simulink model "transientStability_R2014B_SLX"  (R2014b)
settings: Solver=ode4  SolverMode=SingleTasking  StartTime=0.0  StopTime=10  FixedStep=0.01  MaxStep=0.01  RelTol=1e-3  AbsTol=1e-2
undefined symbols (not defined in the file): j, mpc
(part 3 of 4)

== system transientStability_R2014B_SLX/Turbine system/Sped Gov_Hydro Turbine/DEMUXg2 ==
  In1 : Inport
  Dummy Zeros : Constant  Value=zeros(1,mpc.dynamicdata.extraVariables.nb-size(mpc.dynamicdata.turb_hydro,1))
  Mux1 : Mux  Inputs="[mpc.dynamicdata.extraVariables.nb-size(mpc.dynamicdata.turb_hydro,1)  size(mpc.dynamicdata.turb_hydro,1)]"
  Selector4 : Selector  InputPortWidth=mpc.dynamicdata.extraVariables.nb  IndexOptions=Index vector (dialog)  Indices=mpc.dynamicdata.gen_turbineParameters.hydro_turbineParameters.order_hydro  OutputSizes=1
  Out1 : Outport
  wires:
  Mux1/1 -> Selector4/1
  Dummy Zeros/1 -> Mux1/1
  Selector4/1 -> Out1/1
  In1/1 -> Mux1/2

== system transientStability_R2014B_SLX/Turbine system/Sped Gov_Hydro Turbine/Governer ==
  del WB : Inport
  Constant : Constant  Value=mpc.dynamicdata.gen_turbineParameters.hydro_turbineParameters.Pgv_ht0
  Gain : Gain  Gain=1-mpc.dynamicdata.gen_turbineParameters.hydro_turbineParameters.T2_ht./mpc.dynamicdata.gen_turbineParameters.hydro_turbineParameters.T1_ht  SaturateOnIntegerOverflow=on  OutDataTypeStr=Inherit: Same as input  ParamDataTypeStr=Inherit: Same as input
  Gain1 : Gain  Gain=1./mpc.dynamicdata.gen_turbineParameters.hydro_turbineParameters.T1_ht  SaturateOnIntegerOverflow=on  OutDataTypeStr=Inherit: Same as input  ParamDataTypeStr=Inherit: Same as input
  Gain2 : Gain  Gain=mpc.dynamicdata.gen_turbineParameters.hydro_turbineParameters.T2_ht./mpc.dynamicdata.gen_turbineParameters.hydro_turbineParameters.T1_ht  SaturateOnIntegerOverflow=on  OutDataTypeStr=Inherit: Same as input  ParamDataTypeStr=Inherit: Same as input
  Gain3 : Gain  Gain=mpc.dynamicdata.gen_turbineParameters.hydro_turbineParameters.K_ht  SaturateOnIntegerOverflow=on  OutDataTypeStr=Inherit: Same as input  ParamDataTypeStr=Inherit: Same as input
  Gain4 : Gain  Gain=1./mpc.dynamicdata.gen_turbineParameters.hydro_turbineParameters.T3_ht  SaturateOnIntegerOverflow=on  OutDataTypeStr=Inherit: Same as input  ParamDataTypeStr=Inherit: Same as input
  Integrator : Integrator
  Integrator1 : Integrator
  Saturation : Saturate  UpperLimit=mpc.dynamicdata.gen_turbineParameters.hydro_turbineParameters.Pgv_ht_max.*mpc.dynamicdata.gen_turbineParameters.hydro_turbineParameters.Pgv_ht0  LowerLimit=mpc.dynamicdata.gen_turbineParameters.hydro_turbineParameters.Pgv_ht_min.*mpc.dynamicdata.gen_turbineParameters.hydro_turbineParameters.Pgv_ht0
  Sum : Sum  Inputs=+-  SaturateOnIntegerOverflow=on  InputSameDT=on  OutDataTypeStr=Inherit: Same as first input
  Sum1 : Sum  SaturateOnIntegerOverflow=on  InputSameDT=on  OutDataTypeStr=Inherit: Same as first input
  Sum3 : Sum  Inputs=+-  SaturateOnIntegerOverflow=on  InputSameDT=on  OutDataTypeStr=Inherit: Same as first input
  Sum4 : Sum  Inputs=+-  SaturateOnIntegerOverflow=on  InputSameDT=on  OutDataTypeStr=Inherit: Same as first input
  Pgv : Outport
  wires:
  Sum/1 -> Gain1/1
  Gain/1 -> Sum/1
  Integrator/1 -> Sum/2, Sum1/1
  Gain2/1 -> Sum1/2
  Gain1/1 -> Integrator/1
  del WB/1 -> Gain2/1, Gain/1
  Sum1/1 -> Gain3/1
  Gain3/1 -> Sum3/1
  Sum3/1 -> Gain4/1
  Gain4/1 -> Integrator1/1
  Integrator1/1 -> Sum4/2, Sum3/2
  Constant/1 -> Sum4/1
  Sum4/1 -> Saturation/1
  Saturation/1 -> Pgv/1

== system transientStability_R2014B_SLX/Turbine system/Sped Gov_Hydro Turbine/HydroTurbine ==
  Pgv : Inport
  Gain : Gain  Gain=1-(-mpc.dynamicdata.gen_turbineParameters.hydro_turbineParameters.T_wht)./(0.5*mpc.dynamicdata.gen_turbineParameters.hydro_turbineParameters.T_wht)  SaturateOnIntegerOverflow=on  OutDataTypeStr=Inherit: Same as input  ParamDataTypeStr=Inherit: Same as input
  Gain1 : Gain  Gain=1./(0.5*mpc.dynamicdata.gen_turbineParameters.hydro_turbineParameters.T_wht)  SaturateOnIntegerOverflow=on  OutDataTypeStr=Inherit: Same as input  ParamDataTypeStr=Inherit: Same as input
  Gain2 : Gain  Gain=-mpc.dynamicdata.gen_turbineParameters.hydro_turbineParameters.T_wht./(0.5*mpc.dynamicdata.gen_turbineParameters.hydro_turbineParameters.T_wht)  SaturateOnIntegerOverflow=on  OutDataTypeStr=Inherit: Same as input  ParamDataTypeStr=Inherit: Same as input
  Integrator : Integrator  InitialCondition=mpc.dynamicdata.gen_turbineParameters.hydro_turbineParameters.Tgr_ht0
  Sum : Sum  Inputs=+-  SaturateOnIntegerOverflow=on  InputSameDT=on  OutDataTypeStr=Inherit: Same as first input
  Sum1 : Sum  SaturateOnIntegerOverflow=on  InputSameDT=on  OutDataTypeStr=Inherit: Same as first input
  Tm : Outport
  wires:
  Sum1/1 -> Tm/1
  Gain1/1 -> Integrator/1
  Pgv/1 -> Gain2/1, Gain/1
  Gain2/1 -> Sum1/2
  Integrator/1 -> Sum/2, Sum1/1
  Gain/1 -> Sum/1
  Sum/1 -> Gain1/1

== system transientStability_R2014B_SLX/Turbine system/Sped Gov_Hydro Turbine/Select-Turbine ==
  in_1 : Inport
  in_2 : Inport  Port=2
  Switch : Switch  Threshold=1  SaturateOnIntegerOverflow=on  InputSameDT=on
  zeros : Constant  Value=zeros(1,mpc.dynamicdata.extraVariables.nb)
  out_1 : Outport  InitialOutput=0
  wires:
  Switch/1 -> out_1/1
  in_1/1 -> Switch/2
  in_2/1 -> Switch/3
  zeros/1 -> Switch/1

== system transientStability_R2014B_SLX/Turbine system/Speed Gov. Reheat Steam Turbine/DEMUXg2 ==
  In1 : Inport
  Dummy Zeros : Constant  Value=zeros(1,mpc.dynamicdata.extraVariables.nb-size(mpc.dynamicdata.turb_rhst,1))
  Mux1 : Mux  Inputs="[mpc.dynamicdata.extraVariables.nb-size(mpc.dynamicdata.turb_rhst,1)  size(mpc.dynamicdata.turb_rhst,1)]"
  Selector4 : Selector  InputPortWidth=mpc.dynamicdata.extraVariables.nb  IndexOptions=Index vector (dialog)  Indices=mpc.dynamicdata.gen_turbineParameters.Reheat_turbineParameters.order_rhst  OutputSizes=1
  Out1 : Outport
  wires:
  In1/1 -> Mux1/2
  Selector4/1 -> Out1/1
  Dummy Zeros/1 -> Mux1/1
  Mux1/1 -> Selector4/1

== system transientStability_R2014B_SLX/Turbine system/Speed Gov. Reheat Steam Turbine/Governer ==
  dWB : Inport
  Constant : Constant  Value=mpc.dynamicdata.gen_turbineParameters.Reheat_turbineParameters.Pgv_rht0
  Gain : Gain  Gain=1-mpc.dynamicdata.gen_turbineParameters.Reheat_turbineParameters.T2_rht./mpc.dynamicdata.gen_turbineParameters.Reheat_turbineParameters.T1_rht  SaturateOnIntegerOverflow=on  OutDataTypeStr=Inherit: Same as input  ParamDataTypeStr=Inherit: Same as input
  Gain1 : Gain  Gain=1./mpc.dynamicdata.gen_turbineParameters.Reheat_turbineParameters.T1_rht  SaturateOnIntegerOverflow=on  OutDataTypeStr=Inherit: Same as input  ParamDataTypeStr=Inherit: Same as input
  Gain2 : Gain  Gain=mpc.dynamicdata.gen_turbineParameters.Reheat_turbineParameters.T2_rht./mpc.dynamicdata.gen_turbineParameters.Reheat_turbineParameters.T1_rht  SaturateOnIntegerOverflow=on  OutDataTypeStr=Inherit: Same as input  ParamDataTypeStr=Inherit: Same as input
  Gain3 : Gain  Gain=mpc.dynamicdata.gen_turbineParameters.Reheat_turbineParameters.K_rht  SaturateOnIntegerOverflow=on  OutDataTypeStr=Inherit: Same as input  ParamDataTypeStr=Inherit: Same as input
  Gain4 : Gain  Gain=1./mpc.dynamicdata.gen_turbineParameters.Reheat_turbineParameters.T3_rht  SaturateOnIntegerOverflow=on  OutDataTypeStr=Inherit: Same as input  ParamDataTypeStr=Inherit: Same as input
  Integrator : Integrator
  Integrator1 : Integrator  InitialCondition=mpc.dynamicdata.gen_turbineParameters.Reheat_turbineParameters.Pgv_rht0  LimitOutput=on  UpperSaturationLimit=mpc.dynamicdata.gen_turbineParameters.Reheat_turbineParameters.Pgv_rht_max.*mpc.dynamicdata.gen_turbineParameters.Reheat_turbineParameters.Pgv_rht0  LowerSaturationLimit=mpc.dynamicdata.gen_turbineParameters.Reheat_turbineParameters.Pgv_rht_min.*mpc.dynamicdata.gen_turbineParameters.Reheat_turbineParameters.Pgv_rht0
  Sum : Sum  Inputs=+-  SaturateOnIntegerOverflow=on  InputSameDT=on  OutDataTypeStr=Inherit: Same as first input
  Sum1 : Sum  SaturateOnIntegerOverflow=on  InputSameDT=on  OutDataTypeStr=Inherit: Same as first input
  Sum3 : Sum  Inputs=+--  SaturateOnIntegerOverflow=on  InputSameDT=on  OutDataTypeStr=Inherit: Same as first input
  Pgv : Outport
  wires:
  Sum/1 -> Gain1/1
  Gain/1 -> Sum/1
  Integrator/1 -> Sum1/1, Sum/2
  Gain2/1 -> Sum1/2
  Gain1/1 -> Integrator/1
  Sum1/1 -> Gain3/1
  Sum3/1 -> Gain4/1
  Gain4/1 -> Integrator1/1
  Integrator1/1 -> Sum3/3, Pgv/1
  Gain3/1 -> Sum3/2
  Constant/1 -> Sum3/1
  dWB/1 -> Gain/1, Gain2/1

== system transientStability_R2014B_SLX/Turbine system/Speed Gov. Reheat Steam Turbine/Reheat ==
  Pgv : Inport
  Crossover : Subsystem
  Gain3 : Gain  Gain=mpc.dynamicdata.gen_turbineParameters.Reheat_turbineParameters.FHP_rht  SaturateOnIntegerOverflow=on  OutDataTypeStr=Inherit: Same as input  ParamDataTypeStr=Inherit: Same as input
  Gain4 : Gain  Gain=mpc.dynamicdata.gen_turbineParameters.Reheat_turbineParameters.FIP_rht  SaturateOnIntegerOverflow=on  OutDataTypeStr=Inherit: Same as input  ParamDataTypeStr=Inherit: Same as input
  Gain5 : Gain  Gain=mpc.dynamicdata.gen_turbineParameters.Reheat_turbineParameters.FLP_rht  SaturateOnIntegerOverflow=on  OutDataTypeStr=Inherit: Same as input  ParamDataTypeStr=Inherit: Same as input
  Reheater : Subsystem
  St.Chest : Subsystem
  Sum5 : Sum  Inputs=+++  SaturateOnIntegerOverflow=on  InputSameDT=on  OutDataTypeStr=Inherit: Same as first input
  Pm : Outport
  wires:
  Crossover/1(Out1) -> Gain5/1
  Reheater/1(Out1) -> Crossover/1(In1), Gain4/1
  St.Chest/1(Out1) -> Reheater/1(In1), Gain3/1
  Gain5/1 -> Sum5/3
  Gain4/1 -> Sum5/2
  Gain3/1 -> Sum5/1
  Sum5/1 -> Pm/1
  Pgv/1 -> St.Chest/1(In1)

== system transientStability_R2014B_SLX/Turbine system/Speed Gov. Reheat Steam Turbine/Select-Turbine ==
  in_1 : Inport
  in_2 : Inport  Port=2
  Switch : Switch  Threshold=1  SaturateOnIntegerOverflow=on  InputSameDT=on
  zeros : Constant  Value=zeros(1,mpc.dynamicdata.extraVariables.nb)
  out_1 : Outport  InitialOutput=0
  wires:
  Switch/1 -> out_1/1
  in_1/1 -> Switch/2
  in_2/1 -> Switch/3
  zeros/1 -> Switch/1

== system transientStability_R2014B_SLX/Excitation system/Exciter_AC1A /Exciter AC1A/ESS ==
  vfe : Inport
  Gain3 : Gain  Gain=1./mpc.dynamicdata.gen_exciterParameters.AC1A_exciterParameters.TF_AC1A  SaturateOnIntegerOverflow=on  OutDataTypeStr=Inherit: Same as input  ParamDataTypeStr=Inherit: Same as input
  Gain4 : Gain  Gain=mpc.dynamicdata.gen_exciterParameters.AC1A_exciterParameters.KF_AC1A  SaturateOnIntegerOverflow=on  OutDataTypeStr=Inherit: Same as input  ParamDataTypeStr=Inherit: Same as input
  Integrator4 : Integrator  InitialCondition=mpc.dynamicdata.gen_exciterParameters.AC1A_exciterParameters.Fst0_AC1A
  Sum3 : Sum  Inputs=+-  SaturateOnIntegerOverflow=on  InputSameDT=on  OutDataTypeStr=Inherit: Same as first input
  VF1 : Outport
  wires:
  vfe/1 -> Gain4/1
  Sum3/1 -> Gain3/1
  Gain4/1 -> Sum3/1
  Gain3/1 -> Integrator4/1, VF1/1
  Integrator4/1 -> Sum3/2

== system transientStability_R2014B_SLX/Excitation system/Exciter_AC1A /Exciter AC1A/Regulator ==
  Vin : Inport
  Gain : Gain  Gain=1./mpc.dynamicdata.gen_exciterParameters.AC1A_exciterParameters.TA_AC1A  SaturateOnIntegerOverflow=on  OutDataTypeStr=Inherit: Same as input  ParamDataTypeStr=Inherit: Same as input
  Gain1 : Gain  Gain=mpc.dynamicdata.gen_exciterParameters.AC1A_exciterParameters.kA_AC1A  SaturateOnIntegerOverflow=on  OutDataTypeStr=Inherit: Same as input  ParamDataTypeStr=Inherit: Same as input
  Integrator2 : Integrator  InitialCondition=mpc.dynamicdata.gen_exciterParameters.AC1A_exciterParameters.VR0_AC1A  LimitOutput=on  UpperSaturationLimit=mpc.dynamicdata.gen_exciterParameters.AC1A_exciterParameters.VAmax_AC1A  LowerSaturationLimit=mpc.dynamicdata.gen_exciterParameters.AC1A_exciterParameters.VAmin_AC1A
  Sum : Sum  Inputs=+-  SaturateOnIntegerOverflow=on  InputSameDT=on  OutDataTypeStr=Inherit: Same as first input
  VR : Outport
  wires:
  Sum/1 -> Gain/1
  Integrator2/1 -> VR/1, Sum/2
  Gain1/1 -> Sum/1
  Gain/1 -> Integrator2/1
  Vin/1 -> Gain1/1

== system transientStability_R2014B_SLX/Excitation system/Exciter_AC1A /Exciter AC1A/Subsystem1 ==
  VE : Inport
  IFD : Inport  Port=2
  Rec-Reg Curve : Subsystem
  Saturation : Subsystem
  FEX : Outport
  VFE : Outport  Port=2
  wires:
  Rec-Reg Curve/1(Fex) -> FEX/1
  Saturation/1(Vfe) -> VFE/1
  VE/1 -> Saturation/1(Ve), Rec-Reg Curve/2(Ve)
  IFD/1 -> Saturation/2(Ifd), Rec-Reg Curve/1(Ifd)

== system transientStability_R2014B_SLX/Excitation system/Exciter_AC1A /Exciter AC1A/TGR ==
  Ver : Inport
  Gain3 : Gain  Gain=1./mpc.dynamicdata.gen_exciterParameters.AC1A_exciterParameters.TB_AC1A  SaturateOnIntegerOverflow=on  OutDataTypeStr=Inherit: Same as input  ParamDataTypeStr=Inherit: Same as input
  Gain4 : Gain  Gain=mpc.dynamicdata.gen_exciterParameters.AC1A_exciterParameters.TC_AC1A./mpc.dynamicdata.gen_exciterParameters.AC1A_exciterParameters.TB_AC1A  SaturateOnIntegerOverflow=on  OutDataTypeStr=Inherit: Same as input  ParamDataTypeStr=Inherit: Same as input
  Gain5 : Gain  Gain=1-mpc.dynamicdata.gen_exciterParameters.AC1A_exciterParameters.TC_AC1A./mpc.dynamicdata.gen_exciterParameters.AC1A_exciterParameters.TB_AC1A  SaturateOnIntegerOverflow=on  OutDataTypeStr=Inherit: Same as input  ParamDataTypeStr=Inherit: Same as input
  Integrator4 : Integrator  InitialCondition=mpc.dynamicdata.gen_exciterParameters.AC1A_exciterParameters.Tgr0_AC1A
  Sum3 : Sum  SaturateOnIntegerOverflow=on  InputSameDT=on  OutDataTypeStr=Inherit: Same as first input
  Sum4 : Sum  Inputs=+-  SaturateOnIntegerOverflow=on  InputSameDT=on  OutDataTypeStr=Inherit: Same as first input
  Vtgr : Outport
  wires:
  Sum3/1 -> Vtgr/1
  Gain4/1 -> Sum3/2
  Integrator4/1 -> Sum3/1, Sum4/2
  Sum4/1 -> Gain3/1
  Gain5/1 -> Sum4/1
  Gain3/1 -> Integrator4/1
  Ver/1 -> Gain4/1, Gain5/1

== system transientStability_R2014B_SLX/Excitation system/Exciter_AC1A /Exciter AC1A/delay1 ==
  Vin : Inport
  Gain : Gain  Gain=1./mpc.dynamicdata.gen_exciterParameters.AC1A_exciterParameters.Tr_AC1A  SaturateOnIntegerOverflow=on  OutDataTypeStr=Inherit: Same as input  ParamDataTypeStr=Inherit: Same as input
  Integrator2 : Integrator  InitialCondition=mpc.dynamicdata.extraVariables.lfl(mpc.dynamicdata.exc_AC1A(:,1),2)
  Sum : Sum  Inputs=+-  SaturateOnIntegerOverflow=on  InputSameDT=on  OutDataTypeStr=Inherit: Same as first input
  Out1 : Outport
  wires:
  Vin/1 -> Sum/1
  Integrator2/1 -> Sum/2, Out1/1
  Sum/1 -> Gain/1
  Gain/1 -> Integrator2/1

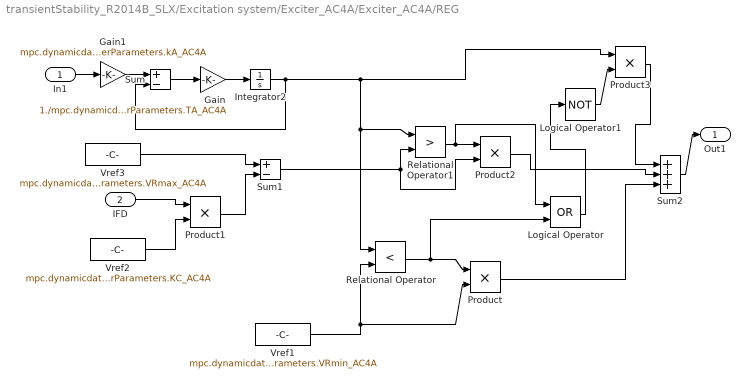
== system transientStability_R2014B_SLX/Excitation system/Exciter_AC4A/Exciter_AC4A/REG ==
  In1 : Inport
  IFD : Inport  Port=2
  Gain : Gain  Gain=1./mpc.dynamicdata.gen_exciterParameters.AC4A_exciterParameters.TA_AC4A  SaturateOnIntegerOverflow=on  OutDataTypeStr=Inherit: Same as input  ParamDataTypeStr=Inherit: Same as input
  Gain1 : Gain  Gain=mpc.dynamicdata.gen_exciterParameters.AC4A_exciterParameters.kA_AC4A  SaturateOnIntegerOverflow=on  OutDataTypeStr=Inherit: Same as input  ParamDataTypeStr=Inherit: Same as input
  Integrator2 : Integrator  InitialCondition=mpc.dynamicdata.gen_exciterParameters.AC4A_exciterParameters.Efd0_AC4A
  Logical Operator : Logic  Operator=OR
  Logical Operator1 : Logic  Operator=NOT
  Product{,1..3} (4 alike) : Product  SaturateOnIntegerOverflow=on  RndMeth=Zero  InputSameDT=on  OutDataTypeStr=Inherit: Same as first input
  Relational Operator : RelationalOperator  Operator=<  InputSameDT=on
  Relational Operator1 : RelationalOperator  Operator=>  InputSameDT=on
  Sum : Sum  Inputs=+-  SaturateOnIntegerOverflow=on  InputSameDT=on  OutDataTypeStr=Inherit: Same as first input
  Sum1 : Sum  Inputs=+-  SaturateOnIntegerOverflow=on  InputSameDT=on  OutDataTypeStr=Inherit: Same as first input
  Sum2 : Sum  Inputs=+++  SaturateOnIntegerOverflow=on  InputSameDT=on  OutDataTypeStr=Inherit: Same as first input
  Vref1 : Constant  Value=mpc.dynamicdata.gen_exciterParameters.AC4A_exciterParameters.VRmin_AC4A
  Vref2 : Constant  Value=mpc.dynamicdata.gen_exciterParameters.AC4A_exciterParameters.KC_AC4A
  Vref3 : Constant  Value=mpc.dynamicdata.gen_exciterParameters.AC4A_exciterParameters.VRmax_AC4A
  Out1 : Outport
  wires:
  In1/1 -> Gain1/1
  Gain1/1 -> Sum/1
  Sum/1 -> Gain/1
  Integrator2/1 -> Sum/2, Relational Operator/1, Relational Operator1/1, Product3/1
  Gain/1 -> Integrator2/1
  Vref1/1 -> Relational Operator/2, Product/2
  Vref2/1 -> Product1/2
  IFD/1 -> Product1/1
  Vref3/1 -> Sum1/1
  Product1/1 -> Sum1/2
  Sum1/1 -> Relational Operator1/2, Product2/2
  Product2/1 -> Sum2/2
  Product/1 -> Sum2/3
  Relational Operator/1 -> Product/1, Logical Operator/2
  Relational Operator1/1 -> Product2/1, Logical Operator/1
  Logical Operator/1 -> Logical Operator1/1
  Logical Operator1/1 -> Product3/2
  Product3/1 -> Sum2/1
  Sum2/1 -> Out1/1

== system transientStability_R2014B_SLX/Excitation system/Exciter_AC4A/Exciter_AC4A/TGR ==
  Ver : Inport
  Gain3 : Gain  Gain=1./mpc.dynamicdata.gen_exciterParameters.AC4A_exciterParameters.TB_AC4A  SaturateOnIntegerOverflow=on  OutDataTypeStr=Inherit: Same as input  ParamDataTypeStr=Inherit: Same as input
  Gain4 : Gain  Gain=mpc.dynamicdata.gen_exciterParameters.AC4A_exciterParameters.TC_AC4A./mpc.dynamicdata.gen_exciterParameters.AC4A_exciterParameters.TB_AC4A  SaturateOnIntegerOverflow=on  OutDataTypeStr=Inherit: Same as input  ParamDataTypeStr=Inherit: Same as input
  Gain5 : Gain  Gain=1-mpc.dynamicdata.gen_exciterParameters.AC4A_exciterParameters.TC_AC4A./mpc.dynamicdata.gen_exciterParameters.AC4A_exciterParameters.TB_AC4A  SaturateOnIntegerOverflow=on  OutDataTypeStr=Inherit: Same as input  ParamDataTypeStr=Inherit: Same as input
  Integrator4 : Integrator  InitialCondition=mpc.dynamicdata.gen_exciterParameters.AC4A_exciterParameters.Tgr0_AC4A
  Sum3 : Sum  SaturateOnIntegerOverflow=on  InputSameDT=on  OutDataTypeStr=Inherit: Same as first input
  Sum4 : Sum  Inputs=+-  SaturateOnIntegerOverflow=on  InputSameDT=on  OutDataTypeStr=Inherit: Same as first input
  V3 : Outport
  wires:
  Gain5/1 -> Sum4/1
  Sum4/1 -> Gain3/1
  Gain3/1 -> Integrator4/1
  Integrator4/1 -> Sum4/2, Sum3/1
  Gain4/1 -> Sum3/2
  Ver/1 -> Gain5/1, Gain4/1
  Sum3/1 -> V3/1

== system transientStability_R2014B_SLX/Excitation system/Exciter_AC4A/Exciter_AC4A/delay1 ==
  Vin : Inport
  Gain : Gain  Gain=1./mpc.dynamicdata.gen_exciterParameters.AC4A_exciterParameters.Tr_AC4A  SaturateOnIntegerOverflow=on  OutDataTypeStr=Inherit: Same as input  ParamDataTypeStr=Inherit: Same as input
  Integrator2 : Integrator  InitialCondition=mpc.dynamicdata.extraVariables.lfl(mpc.dynamicdata.exc_AC4A(:,1),2)
  Sum : Sum  Inputs=+-  SaturateOnIntegerOverflow=on  InputSameDT=on  OutDataTypeStr=Inherit: Same as first input
  Out1 : Outport
  wires:
  Vin/1 -> Sum/1
  Integrator2/1 -> Sum/2, Out1/1
  Sum/1 -> Gain/1
  Gain/1 -> Integrator2/1

== system transientStability_R2014B_SLX/Excitation system/Exciter_DC1A/Subsystem/ESS ==
  Efd : Inport
  Gain3 : Gain  Gain=1./mpc.dynamicdata.gen_exciterParameters.DC1A_exciterParameters.TF_DC1A  SaturateOnIntegerOverflow=on  OutDataTypeStr=Inherit: Same as input  ParamDataTypeStr=Inherit: Same as input
  Gain4 : Gain  Gain=mpc.dynamicdata.gen_exciterParameters.DC1A_exciterParameters.KF_DC1A  SaturateOnIntegerOverflow=on  OutDataTypeStr=Inherit: Same as input  ParamDataTypeStr=Inherit: Same as input
  Integrator4 : Integrator  InitialCondition=mpc.dynamicdata.gen_exciterParameters.DC1A_exciterParameters.Fst0_DC1A
  Sum3 : Sum  Inputs=+-  SaturateOnIntegerOverflow=on  InputSameDT=on  OutDataTypeStr=Inherit: Same as first input
  VF : Outport
  wires:
  Gain4/1 -> Sum3/1
  Sum3/1 -> Gain3/1
  Integrator4/1 -> Sum3/2
  Gain3/1 -> Integrator4/1, VF/1
  Efd/1 -> Gain4/1

== system transientStability_R2014B_SLX/Excitation system/Exciter_DC1A/Subsystem/Regulator ==
  Vin : Inport
  Gain : Gain  Gain=1./mpc.dynamicdata.gen_exciterParameters.DC1A_exciterParameters.TA_DC1A  SaturateOnIntegerOverflow=on  OutDataTypeStr=Inherit: Same as input  ParamDataTypeStr=Inherit: Same as input
  Gain1 : Gain  Gain=mpc.dynamicdata.gen_exciterParameters.DC1A_exciterParameters.KA_DC1A  SaturateOnIntegerOverflow=on  OutDataTypeStr=Inherit: Same as input  ParamDataTypeStr=Inherit: Same as input
  Integrator2 : Integrator  InitialCondition=mpc.dynamicdata.gen_exciterParameters.DC1A_exciterParameters.VR0_DC1A  LimitOutput=on  UpperSaturationLimit=mpc.dynamicdata.gen_exciterParameters.DC1A_exciterParameters.VRmax_DC1A  LowerSaturationLimit=mpc.dynamicdata.gen_exciterParameters.DC1A_exciterParameters.VRmin_DC1A
  Sum : Sum  Inputs=+-  SaturateOnIntegerOverflow=on  InputSameDT=on  OutDataTypeStr=Inherit: Same as first input
  Out1 : Outport
  wires:
  Gain1/1 -> Sum/1
  Integrator2/1 -> Sum/2, Out1/1
  Sum/1 -> Gain/1
  Gain/1 -> Integrator2/1
  Vin/1 -> Gain1/1

== system transientStability_R2014B_SLX/Excitation system/Exciter_DC1A/Subsystem/Saturation ==
  Efd : Inport
  Constant : Constant  Value=mpc.dynamicdata.gen_exciterParameters.DC1A_exciterParameters.B_DC1A
  Constant1 : Constant  Value=mpc.dynamicdata.gen_exciterParameters.DC1A_exciterParameters.A_DC1A
  Constant2 : Constant  Value=mpc.dynamicdata.gen_exciterParameters.DC1A_exciterParameters.KE_DC1A
  Math Function : Math  SaturateOnIntegerOverflow=on
  Product : Product  SaturateOnIntegerOverflow=on  RndMeth=Zero  InputSameDT=on  OutDataTypeStr=Inherit: Same as first input
  Product1 : Product  SaturateOnIntegerOverflow=on  RndMeth=Zero  InputSameDT=on  OutDataTypeStr=Inherit: Same as first input
  Product2 : Product  SaturateOnIntegerOverflow=on  RndMeth=Zero  InputSameDT=on  OutDataTypeStr=Inherit: Same as first input
  Sum2 : Sum  SaturateOnIntegerOverflow=on  InputSameDT=on  OutDataTypeStr=Inherit: Same as first input
  VRb : Outport
  wires:
  Constant/1 -> Product/1
  Product/1 -> Math Function/1
  Math Function/1 -> Product1/1
  Constant1/1 -> Product1/2
  Product1/1 -> Sum2/1
  Constant2/1 -> Sum2/2
  Sum2/1 -> Product2/1
  Efd/1 -> Product/2, Product2/2
  Product2/1 -> VRb/1

== system transientStability_R2014B_SLX/Excitation system/Exciter_DC1A/Subsystem/TGR ==
  Ver : Inport
  Gain3 : Gain  Gain=1./mpc.dynamicdata.gen_exciterParameters.DC1A_exciterParameters.TB_DC1A  SaturateOnIntegerOverflow=on  OutDataTypeStr=Inherit: Same as input  ParamDataTypeStr=Inherit: Same as input
  Gain4 : Gain  Gain=mpc.dynamicdata.gen_exciterParameters.DC1A_exciterParameters.TC_DC1A./mpc.dynamicdata.gen_exciterParameters.DC1A_exciterParameters.TB_DC1A  SaturateOnIntegerOverflow=on  OutDataTypeStr=Inherit: Same as input  ParamDataTypeStr=Inherit: Same as input
  Gain5 : Gain  Gain=1-mpc.dynamicdata.gen_exciterParameters.DC1A_exciterParameters.TC_DC1A./mpc.dynamicdata.gen_exciterParameters.DC1A_exciterParameters.TB_DC1A  SaturateOnIntegerOverflow=on  OutDataTypeStr=Inherit: Same as input  ParamDataTypeStr=Inherit: Same as input
  Integrator4 : Integrator  InitialCondition=mpc.dynamicdata.gen_exciterParameters.DC1A_exciterParameters.Tgr0_DC1A
  Sum3 : Sum  SaturateOnIntegerOverflow=on  InputSameDT=on  OutDataTypeStr=Inherit: Same as first input
  Sum4 : Sum  Inputs=+-  SaturateOnIntegerOverflow=on  InputSameDT=on  OutDataTypeStr=Inherit: Same as first input
  V3 : Outport
  wires:
  Gain5/1 -> Sum4/1
  Sum4/1 -> Gain3/1
  Gain3/1 -> Integrator4/1
  Integrator4/1 -> Sum4/2, Sum3/1
  Gain4/1 -> Sum3/2
  Ver/1 -> Gain5/1, Gain4/1
  Sum3/1 -> V3/1

== system transientStability_R2014B_SLX/Excitation system/Exciter_DC1A/Subsystem/delay1 ==
  Vin : Inport
  Gain : Gain  Gain=1./mpc.dynamicdata.gen_exciterParameters.DC1A_exciterParameters.Tr_DC1A  SaturateOnIntegerOverflow=on  OutDataTypeStr=Inherit: Same as input  ParamDataTypeStr=Inherit: Same as input
  Integrator2 : Integrator  InitialCondition=mpc.dynamicdata.extraVariables.lfl(mpc.dynamicdata.exc_DC1A(:,1),2)
  Sum : Sum  Inputs=+-  SaturateOnIntegerOverflow=on  InputSameDT=on  OutDataTypeStr=Inherit: Same as first input
  Out1 : Outport
  wires:
  Vin/1 -> Sum/1
  Integrator2/1 -> Sum/2, Out1/1
  Sum/1 -> Gain/1
  Gain/1 -> Integrator2/1

== system transientStability_R2014B_SLX/Excitation system/Exciter_ST1A/exc_ST1A/ESS ==
  Efd : Inport
  Gain3 : Gain  Gain=1./mpc.dynamicdata.gen_exciterParameters.ST1A_exciterParameters.TF_ST1A  SaturateOnIntegerOverflow=on  OutDataTypeStr=Inherit: Same as input  ParamDataTypeStr=Inherit: Same as input
  Gain4 : Gain  Gain=mpc.dynamicdata.gen_exciterParameters.ST1A_exciterParameters.KF_ST1A  SaturateOnIntegerOverflow=on  OutDataTypeStr=Inherit: Same as input  ParamDataTypeStr=Inherit: Same as input
  Integrator4 : Integrator  InitialCondition=mpc.dynamicdata.gen_exciterParameters.ST1A_exciterParameters.Fst0_ST1A
  Sum3 : Sum  Inputs=+-  SaturateOnIntegerOverflow=on  InputSameDT=on  OutDataTypeStr=Inherit: Same as first input
  VF : Outport
  wires:
  Gain4/1 -> Sum3/1
  Sum3/1 -> Gain3/1
  Integrator4/1 -> Sum3/2
  Gain3/1 -> Integrator4/1, VF/1
  Efd/1 -> Gain4/1

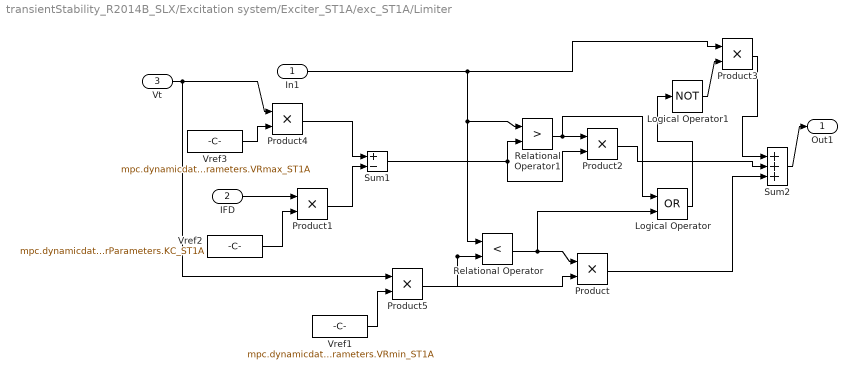
== system transientStability_R2014B_SLX/Excitation system/Exciter_ST1A/exc_ST1A/Limiter ==
  In1 : Inport
  IFD : Inport  Port=2
  Vt : Inport  Port=3
  Logical Operator : Logic  Operator=OR
  Logical Operator1 : Logic  Operator=NOT
  Product{,1..5} (6 alike) : Product  SaturateOnIntegerOverflow=on  RndMeth=Zero  InputSameDT=on  OutDataTypeStr=Inherit: Same as first input
  Relational Operator : RelationalOperator  Operator=<  InputSameDT=on
  Relational Operator1 : RelationalOperator  Operator=>  InputSameDT=on
  Sum1 : Sum  Inputs=+-  SaturateOnIntegerOverflow=on  InputSameDT=on  OutDataTypeStr=Inherit: Same as first input
  Sum2 : Sum  Inputs=+++  SaturateOnIntegerOverflow=on  InputSameDT=on  OutDataTypeStr=Inherit: Same as first input
  Vref1 : Constant  Value=mpc.dynamicdata.gen_exciterParameters.ST1A_exciterParameters.VRmin_ST1A
  Vref2 : Constant  Value=mpc.dynamicdata.gen_exciterParameters.ST1A_exciterParameters.KC_ST1A
  Vref3 : Constant  Value=mpc.dynamicdata.gen_exciterParameters.ST1A_exciterParameters.VRmax_ST1A
  Out1 : Outport
  wires:
  Vref2/1 -> Product1/2
  IFD/1 -> Product1/1
  Product1/1 -> Sum1/2
  Sum1/1 -> Relational Operator1/2, Product2/2
  Product2/1 -> Sum2/2
  Product/1 -> Sum2/3
  Relational Operator/1 -> Product/1, Logical Operator/2
  Relational Operator1/1 -> Product2/1, Logical Operator/1
  Logical Operator/1 -> Logical Operator1/1
  Logical Operator1/1 -> Product3/2
  Product3/1 -> Sum2/1
  Sum2/1 -> Out1/1
  In1/1 -> Relational Operator/1, Relational Operator1/1, Product3/1
  Vref3/1 -> Product4/2
  Product4/1 -> Sum1/1
  Vt/1 -> Product4/1, Product5/1
  Product5/1 -> Relational Operator/2, Product/2
  Vref1/1 -> Product5/2

== system transientStability_R2014B_SLX/Excitation system/Exciter_ST1A/exc_ST1A/Rergulator ==
  In1 : Inport
  Gain : Gain  Gain=1./mpc.dynamicdata.gen_exciterParameters.ST1A_exciterParameters.TA_ST1A  SaturateOnIntegerOverflow=on  OutDataTypeStr=Inherit: Same as input  ParamDataTypeStr=Inherit: Same as input
  Gain1 : Gain  Gain=mpc.dynamicdata.gen_exciterParameters.ST1A_exciterParameters.kA_ST1A  SaturateOnIntegerOverflow=on  OutDataTypeStr=Inherit: Same as input  ParamDataTypeStr=Inherit: Same as input
  Integrator2 : Integrator  InitialCondition=mpc.dynamicdata.gen_exciterParameters.ST1A_exciterParameters.Efd0_ST1A
  Sum : Sum  Inputs=+-  SaturateOnIntegerOverflow=on  InputSameDT=on  OutDataTypeStr=Inherit: Same as first input
  Out1 : Outport
  wires:
  Gain/1 -> Integrator2/1
  Sum/1 -> Gain/1
  Gain1/1 -> Sum/1
  Integrator2/1 -> Sum/2, Out1/1
  In1/1 -> Gain1/1

== system transientStability_R2014B_SLX/Excitation system/Exciter_ST1A/exc_ST1A/TGR ==
  Ver : Inport
  Gain3 : Gain  Gain=1./mpc.dynamicdata.gen_exciterParameters.ST1A_exciterParameters.TB_ST1A  SaturateOnIntegerOverflow=on  OutDataTypeStr=Inherit: Same as input  ParamDataTypeStr=Inherit: Same as input
  Gain4 : Gain  Gain=mpc.dynamicdata.gen_exciterParameters.ST1A_exciterParameters.TC_ST1A./mpc.dynamicdata.gen_exciterParameters.ST1A_exciterParameters.TB_ST1A  SaturateOnIntegerOverflow=on  OutDataTypeStr=Inherit: Same as input  ParamDataTypeStr=Inherit: Same as input
  Gain5 : Gain  Gain=1-mpc.dynamicdata.gen_exciterParameters.ST1A_exciterParameters.TC_ST1A./mpc.dynamicdata.gen_exciterParameters.ST1A_exciterParameters.TB_ST1A  SaturateOnIntegerOverflow=on  OutDataTypeStr=Inherit: Same as input  ParamDataTypeStr=Inherit: Same as input
  Integrator4 : Integrator  InitialCondition=mpc.dynamicdata.gen_exciterParameters.ST1A_exciterParameters.Tgr0_ST1A
  Sum3 : Sum  SaturateOnIntegerOverflow=on  InputSameDT=on  OutDataTypeStr=Inherit: Same as first input
  Sum4 : Sum  Inputs=+-  SaturateOnIntegerOverflow=on  InputSameDT=on  OutDataTypeStr=Inherit: Same as first input
  V3 : Outport
  wires:
  Gain5/1 -> Sum4/1
  Sum4/1 -> Gain3/1
  Gain3/1 -> Integrator4/1
  Integrator4/1 -> Sum4/2, Sum3/1
  Gain4/1 -> Sum3/2
  Ver/1 -> Gain5/1, Gain4/1
  Sum3/1 -> V3/1

== system transientStability_R2014B_SLX/Excitation system/Exciter_ST2A/ST2A_Exciter/ESS ==
  EFD : Inport
  Gain3 : Gain  Gain=1./mpc.dynamicdata.gen_exciterParameters.ST2A_exciterParameters.TF_ST2A  SaturateOnIntegerOverflow=on  OutDataTypeStr=Inherit: Same as input  ParamDataTypeStr=Inherit: Same as input
  Gain4 : Gain  Gain=mpc.dynamicdata.gen_exciterParameters.ST2A_exciterParameters.KF_ST2A  SaturateOnIntegerOverflow=on  OutDataTypeStr=Inherit: Same as input  ParamDataTypeStr=Inherit: Same as input
  Integrator4 : Integrator  InitialCondition=mpc.dynamicdata.gen_exciterParameters.ST2A_exciterParameters.Fst0_ST2A
  Sum3 : Sum  Inputs=+-  SaturateOnIntegerOverflow=on  InputSameDT=on  OutDataTypeStr=Inherit: Same as first input
  VF : Outport
  wires:
  EFD/1 -> Gain4/1
  Gain3/1 -> VF/1, Integrator4/1
  Integrator4/1 -> Sum3/2
  Sum3/1 -> Gain3/1
  Gain4/1 -> Sum3/1

== system transientStability_R2014B_SLX/Excitation system/Exciter_ST2A/ST2A_Exciter/Regulator ==
  Vin : Inport
  Gain : Gain  Gain=1./mpc.dynamicdata.gen_exciterParameters.ST2A_exciterParameters.TA_ST2A  SaturateOnIntegerOverflow=on  OutDataTypeStr=Inherit: Same as input  ParamDataTypeStr=Inherit: Same as input
  Gain1 : Gain  Gain=mpc.dynamicdata.gen_exciterParameters.ST2A_exciterParameters.kA_ST2A  SaturateOnIntegerOverflow=on  OutDataTypeStr=Inherit: Same as input  ParamDataTypeStr=Inherit: Same as input
  Integrator2 : Integrator  InitialCondition=mpc.dynamicdata.gen_exciterParameters.ST2A_exciterParameters.VR0_ST2A  LimitOutput=on  UpperSaturationLimit=mpc.dynamicdata.gen_exciterParameters.ST2A_exciterParameters.VRmax_ST2A  LowerSaturationLimit=mpc.dynamicdata.gen_exciterParameters.ST2A_exciterParameters.VRmin_ST2A
  Sum : Sum  Inputs=+-  SaturateOnIntegerOverflow=on  InputSameDT=on  OutDataTypeStr=Inherit: Same as first input
  Out1 : Outport
  wires:
  Vin/1 -> Gain1/1
  Gain/1 -> Integrator2/1
  Sum/1 -> Gain/1
  Integrator2/1 -> Out1/1, Sum/2
  Gain1/1 -> Sum/1

== system transientStability_R2014B_SLX/Excitation system/Exciter_ST2A/ST2A_Exciter/Subsystem ==
  VT : Inport
  "IFD " : Inport  Port=2
  Ia : Inport  Port=3
  Product3 : Product  SaturateOnIntegerOverflow=on  RndMeth=Zero  InputSameDT=on  OutDataTypeStr=Inherit: Same as first input
  Subsystem : Subsystem
  Subsystem2 : Subsystem
  VB : Outport
  wires:
  VT/1 -> Subsystem/1(VT)
  Subsystem/1(VE) -> Subsystem2/2(VE), Product3/1
  Ia/1 -> Subsystem/2(Ia)
  "IFD "/1 -> Subsystem2/1(IFD)
  Product3/1 -> VB/1
  Subsystem2/1(Fex) -> Product3/2

== system transientStability_R2014B_SLX/Excitation system/Exciter_ST2A/ST2A_Exciter/exciter ==
  In1 : Inport
  Gain2 : Gain  Gain=1./mpc.dynamicdata.gen_exciterParameters.ST2A_exciterParameters.TE_ST2A  SaturateOnIntegerOverflow=on  OutDataTypeStr=Inherit: Same as input  ParamDataTypeStr=Inherit: Same as input
  Gain3 : Gain  Gain=mpc.dynamicdata.gen_exciterParameters.ST2A_exciterParameters.KE_ST2A  SaturateOnIntegerOverflow=on  OutDataTypeStr=Inherit: Same as input  ParamDataTypeStr=Inherit: Same as input
  Integrator3 : Integrator  InitialCondition=mpc.dynamicdata.gen_exciterParameters.ST2A_exciterParameters.Efd0_ST2A  LimitOutput=on  UpperSaturationLimit=mpc.dynamicdata.gen_exciterParameters.ST2A_exciterParameters.EFDmax_ST2A  LowerSaturationLimit=0
  Sum1 : Sum  Inputs=+-  SaturateOnIntegerOverflow=on  InputSameDT=on  OutDataTypeStr=Inherit: Same as first input
  Out1 : Outport
  wires:
  Gain2/1 -> Integrator3/1
  In1/1 -> Sum1/1
  Sum1/1 -> Gain2/1
  Gain3/1 -> Sum1/2
  Integrator3/1 -> Out1/1, Gain3/1

== system transientStability_R2014B_SLX/PSS/delP_Omega_PSS/Filtering M=2 and N=4/Subsystem ==
  In1 : Inport
  Compensator : Subsystem
  delay1 : Subsystem
  Out2 : Outport
  wires:
  In1/1 -> Compensator/1(in)
  Compensator/1(Vs) -> delay1/1(Vin)
  delay1/1(Out1) -> Out2/1

== system transientStability_R2014B_SLX/PSS/delP_Omega_PSS/Filtering M=2 and N=4/Subsystem1 ==
  In1 : Inport
  Compensator : Subsystem
  delay1 : Subsystem
  Out2 : Outport
  wires:
  delay1/1(Out1) -> Out2/1
  Compensator/1(Vs) -> delay1/1(Vin)
  In1/1 -> Compensator/1(in)

== system transientStability_R2014B_SLX/PSS/delP_Omega_PSS/Filtering M=2 and N=4/Subsystem2 ==
  In1 : Inport
  Compensator : Subsystem
  delay1 : Subsystem
  Out2 : Outport
  wires:
  In1/1 -> Compensator/1(in)
  Compensator/1(Vs) -> delay1/1(Vin)
  delay1/1(Out1) -> Out2/1

== system transientStability_R2014B_SLX/PSS/delP_Omega_PSS/Filtering M=2 and N=4/Subsystem3 ==
  In1 : Inport
  Compensator : Subsystem
  delay1 : Subsystem
  Out2 : Outport
  wires:
  delay1/1(Out1) -> Out2/1
  Compensator/1(Vs) -> delay1/1(Vin)
  In1/1 -> Compensator/1(in)

== system transientStability_R2014B_SLX/PSS/frequency_input_PSS /delta_Freq/derivative1 ==
  In3 : Inport
  1/1+s*Tf : Subsystem
  1/Tf : Gain  Gain=[1./0.02]/2/pi  SaturateOnIntegerOverflow=on  OutDataTypeStr=Inherit: Same as input  ParamDataTypeStr=Inherit: Same as input
  Sum6 : Sum  Inputs=+-  SaturateOnIntegerOverflow=on  InputSameDT=on  OutDataTypeStr=Inherit: Same as first input
  Out2 : Outport
  wires:
  1/Tf/1 -> Out2/1
  Sum6/1 -> 1/Tf/1
  1/1+s*Tf/1(Out1) -> Sum6/2
  In3/1 -> Sum6/1, 1/1+s*Tf/1(In1)

== system transientStability_R2014B_SLX/PSS/frequency_input_PSS /delta_Freq/derivative2 ==
  In3 : Inport
  1/1+s*Tf : Subsystem
  1/Tf : Gain  Gain=[1./0.02]/2/pi  SaturateOnIntegerOverflow=on  OutDataTypeStr=Inherit: Same as input  ParamDataTypeStr=Inherit: Same as input
  Sum6 : Sum  Inputs=+-  SaturateOnIntegerOverflow=on  InputSameDT=on  OutDataTypeStr=Inherit: Same as first input
  Out2 : Outport
  wires:
  In3/1 -> 1/1+s*Tf/1(In1), Sum6/1
  1/1+s*Tf/1(Out1) -> Sum6/2
  Sum6/1 -> 1/Tf/1
  1/Tf/1 -> Out2/1

== system transientStability_R2014B_SLX/STATIC LOADS/delta_Freq/derivative1/1//1+s*Tf ==
  In1 : Inport
  1/Tf : Gain  Gain=[1./0.02]  SaturateOnIntegerOverflow=on  OutDataTypeStr=Inherit: Same as input  ParamDataTypeStr=Inherit: Same as input
  In2 : Integrator  InitialCondition=imag(mpc.dynamicdata.Vpre(mpc.dynamicdata.extraVariables.ld(:,1)))
  Sum3 : Sum  Inputs=+-  SaturateOnIntegerOverflow=on  InputSameDT=on  OutDataTypeStr=Inherit: Same as first input
  Out1 : Outport
  wires:
  Sum3/1 -> 1/Tf/1
  1/Tf/1 -> In2/1
  In2/1 -> Sum3/2, Out1/1
  In1/1 -> Sum3/1

== system transientStability_R2014B_SLX/STATIC LOADS/delta_Freq/derivative2/1//1+s*Tf ==
  In1 : Inport
  1/Tf : Gain  Gain=[1./0.02]  SaturateOnIntegerOverflow=on  OutDataTypeStr=Inherit: Same as input  ParamDataTypeStr=Inherit: Same as input
  In2 : Integrator  InitialCondition=real(mpc.dynamicdata.Vpre(mpc.dynamicdata.extraVariables.ld(:,1)))
  Sum3 : Sum  Inputs=+-  SaturateOnIntegerOverflow=on  InputSameDT=on  OutDataTypeStr=Inherit: Same as first input
  Out1 : Outport
  wires:
  In2/1 -> Out1/1, Sum3/2
  1/Tf/1 -> In2/1
  Sum3/1 -> 1/Tf/1
  In1/1 -> Sum3/1

== system transientStability_R2014B_SLX/Turbine system/Speed Gov. Reheat Steam Turbine/Reheat/Crossover ==
  In1 : Inport
  Gain2 : Gain  Gain=1./mpc.dynamicdata.gen_turbineParameters.Reheat_turbineParameters.TCO_rht  SaturateOnIntegerOverflow=on  OutDataTypeStr=Inherit: Same as input  ParamDataTypeStr=Inherit: Same as input
  Integrator2 : Integrator  InitialCondition=mpc.dynamicdata.gen_turbineParameters.Reheat_turbineParameters.LP_rht0
  Sum2 : Sum  Inputs=|+-  SaturateOnIntegerOverflow=on  InputSameDT=on  OutDataTypeStr=Inherit: Same as first input
  Out1 : Outport
  wires:
  Gain2/1 -> Integrator2/1
  Sum2/1 -> Gain2/1
  Integrator2/1 -> Sum2/2, Out1/1
  In1/1 -> Sum2/1

== system transientStability_R2014B_SLX/Turbine system/Speed Gov. Reheat Steam Turbine/Reheat/Reheater ==
  In1 : Inport
  Gain1 : Gain  Gain=1./mpc.dynamicdata.gen_turbineParameters.Reheat_turbineParameters.TRH_rht  SaturateOnIntegerOverflow=on  OutDataTypeStr=Inherit: Same as input  ParamDataTypeStr=Inherit: Same as input
  Integrator1 : Integrator  InitialCondition=mpc.dynamicdata.gen_turbineParameters.Reheat_turbineParameters.IP_rht0
  Sum1 : Sum  Inputs=|+-  SaturateOnIntegerOverflow=on  InputSameDT=on  OutDataTypeStr=Inherit: Same as first input
  Out1 : Outport
  wires:
  Gain1/1 -> Integrator1/1
  Sum1/1 -> Gain1/1
  Integrator1/1 -> Sum1/2, Out1/1
  In1/1 -> Sum1/1

== system transientStability_R2014B_SLX/Turbine system/Speed Gov. Reheat Steam Turbine/Reheat/St.Chest ==
  In1 : Inport
  Gain : Gain  Gain=1./mpc.dynamicdata.gen_turbineParameters.Reheat_turbineParameters.TCH_rht  SaturateOnIntegerOverflow=on  OutDataTypeStr=Inherit: Same as input  ParamDataTypeStr=Inherit: Same as input
  Integrator : Integrator  InitialCondition=mpc.dynamicdata.gen_turbineParameters.Reheat_turbineParameters.HP_rht0
  Sum : Sum  Inputs=|+-  SaturateOnIntegerOverflow=on  InputSameDT=on  OutDataTypeStr=Inherit: Same as first input
  Out1 : Outport
  wires:
  Gain/1 -> Integrator/1
  Sum/1 -> Gain/1
  Integrator/1 -> Sum/2, Out1/1
  In1/1 -> Sum/1

== system transientStability_R2014B_SLX/Excitation system/Exciter_AC1A /Exciter AC1A/Subsystem1/Rec-Reg Curve ==
  Ifd : Inport
  Ve : Inport  Port=2
  IN : Product  Inputs=*/  SaturateOnIntegerOverflow=on  RndMeth=Zero  InputSameDT=on  OutDataTypeStr=Inherit: Same as first input
  KC_AC1A : Gain  Gain=mpc.dynamicdata.gen_exciterParameters.AC1A_exciterParameters.KC_AC1A  SaturateOnIntegerOverflow=on  OutDataTypeStr=Inherit: Same as input  ParamDataTypeStr=Inherit: Same as input
  "Rec-Reg Eq " : Subsystem
  Fex : Outport
  wires:
  Ve/1 -> IN/2
  IN/1 -> "Rec-Reg Eq "/1(IN)
  Ifd/1 -> KC_AC1A/1
  KC_AC1A/1 -> IN/1
  "Rec-Reg Eq "/1(Fex) -> Fex/1

== system transientStability_R2014B_SLX/Excitation system/Exciter_AC1A /Exciter AC1A/Subsystem1/Saturation ==
  note: KD_AC1A
  Ve : Inport
  Ifd : Inport  Port=2
  Gain2 : Gain  Gain=mpc.dynamicdata.gen_exciterParameters.AC1A_exciterParameters.KD_AC1A  SaturateOnIntegerOverflow=on  OutDataTypeStr=Inherit: Same as input  ParamDataTypeStr=Inherit: Same as input
  Saturation : Subsystem
  Sum : Sum  SaturateOnIntegerOverflow=on  InputSameDT=on  OutDataTypeStr=Inherit: Same as first input
  Vfe : Outport
  wires:
  Ve/1 -> Saturation/1(VE)
  Ifd/1 -> Gain2/1
  Saturation/1(VRb) -> Sum/1
  Gain2/1 -> Sum/2
  Sum/1 -> Vfe/1

== system transientStability_R2014B_SLX/Excitation system/Exciter_ST2A/ST2A_Exciter/Subsystem/Subsystem ==
  VT : Inport
  Ia : Inport  Port=2
  Abs : Abs  SaturateOnIntegerOverflow=on
  Constant : Constant  Value=mpc.dynamicdata.gen_exciterParameters.ST2A_exciterParameters.KP_ST2A
  Constant1 : Constant  Value=j*mpc.dynamicdata.gen_exciterParameters.ST2A_exciterParameters.KI_ST2A
  Product1 : Product  SaturateOnIntegerOverflow=on  RndMeth=Zero  InputSameDT=on  OutDataTypeStr=Inherit: Same as first input
  Product2 : Product  SaturateOnIntegerOverflow=on  RndMeth=Zero  InputSameDT=on  OutDataTypeStr=Inherit: Same as first input
  Sum2 : Sum  SaturateOnIntegerOverflow=on  InputSameDT=on  OutDataTypeStr=Inherit: Same as first input
  VE : Outport
  wires:
  Constant/1 -> Product1/1
  VT/1 -> Product1/2
  Constant1/1 -> Product2/2
  Ia/1 -> Product2/1
  Sum2/1 -> Abs/1
  Product1/1 -> Sum2/1
  Product2/1 -> Sum2/2
  Abs/1 -> VE/1

== system transientStability_R2014B_SLX/Excitation system/Exciter_ST2A/ST2A_Exciter/Subsystem/Subsystem2 ==
  IFD : Inport
  VE : Inport  Port=2
  Gain : Gain  Gain=mpc.dynamicdata.gen_exciterParameters.ST2A_exciterParameters.KC_ST2A  SaturateOnIntegerOverflow=on  OutDataTypeStr=Inherit: Same as input  ParamDataTypeStr=Inherit: Same as input
  Product2 : Product  Inputs=*/  SaturateOnIntegerOverflow=on  RndMeth=Zero  InputSameDT=on  OutDataTypeStr=Inherit: Same as first input
  Subsystem : Subsystem
  Fex : Outport
  wires:
  VE/1 -> Product2/2
  Gain/1 -> Product2/1
  IFD/1 -> Gain/1
  Product2/1 -> Subsystem/1(IN)
  Subsystem/1(Fex) -> Fex/1

== system transientStability_R2014B_SLX/PSS/delP_Omega_PSS/Filtering M=2 and N=4/Subsystem/Compensator ==
  in : Inport
  Gain3 : Gain  Gain=1./mpc.dynamicdata.gen_pssParameters.pss_delPw_signalParameters.T9_delPw  SaturateOnIntegerOverflow=on  OutDataTypeStr=Inherit: Same as input  ParamDataTypeStr=Inherit: Same as input
  Gain4 : Gain  Gain=mpc.dynamicdata.gen_pssParameters.pss_delPw_signalParameters.T8_delPw./mpc.dynamicdata.gen_pssParameters.pss_delPw_signalParameters.T9_delPw  SaturateOnIntegerOverflow=on  OutDataTypeStr=Inherit: Same as input  ParamDataTypeStr=Inherit: Same as input
  Gain5 : Gain  Gain=1-mpc.dynamicdata.gen_pssParameters.pss_delPw_signalParameters.T8_delPw./mpc.dynamicdata.gen_pssParameters.pss_delPw_signalParameters.T9_delPw  SaturateOnIntegerOverflow=on  OutDataTypeStr=Inherit: Same as input  ParamDataTypeStr=Inherit: Same as input
  Integrator4 : Integrator
  Sum3 : Sum  SaturateOnIntegerOverflow=on  InputSameDT=on  OutDataTypeStr=Inherit: Same as first input
  Sum4 : Sum  Inputs=+-  SaturateOnIntegerOverflow=on  InputSameDT=on  OutDataTypeStr=Inherit: Same as first input
  Vs : Outport
  wires:
  Gain5/1 -> Sum4/1
  Sum4/1 -> Gain3/1
  Gain3/1 -> Integrator4/1
  Integrator4/1 -> Sum4/2, Sum3/1
  Gain4/1 -> Sum3/2
  in/1 -> Gain5/1, Gain4/1
  Sum3/1 -> Vs/1

== system transientStability_R2014B_SLX/PSS/delP_Omega_PSS/Filtering M=2 and N=4/Subsystem/delay1 ==
  Vin : Inport
  Gain : Gain  Gain=1./mpc.dynamicdata.gen_pssParameters.pss_delPw_signalParameters.T9_delPw  SaturateOnIntegerOverflow=on  OutDataTypeStr=Inherit: Same as input  ParamDataTypeStr=Inherit: Same as input
  Integrator2 : Integrator
  Sum : Sum  Inputs=+-  SaturateOnIntegerOverflow=on  InputSameDT=on  OutDataTypeStr=Inherit: Same as first input
  Out1 : Outport
  wires:
  Vin/1 -> Sum/1
  Integrator2/1 -> Sum/2, Out1/1
  Sum/1 -> Gain/1
  Gain/1 -> Integrator2/1

== system transientStability_R2014B_SLX/PSS/delP_Omega_PSS/Filtering M=2 and N=4/Subsystem1/Compensator ==
  in : Inport
  Gain3 : Gain  Gain=1./mpc.dynamicdata.gen_pssParameters.pss_delPw_signalParameters.T9_delPw  SaturateOnIntegerOverflow=on  OutDataTypeStr=Inherit: Same as input  ParamDataTypeStr=Inherit: Same as input
  Gain4 : Gain  Gain=mpc.dynamicdata.gen_pssParameters.pss_delPw_signalParameters.T8_delPw./mpc.dynamicdata.gen_pssParameters.pss_delPw_signalParameters.T9_delPw  SaturateOnIntegerOverflow=on  OutDataTypeStr=Inherit: Same as input  ParamDataTypeStr=Inherit: Same as input
  Gain5 : Gain  Gain=1-mpc.dynamicdata.gen_pssParameters.pss_delPw_signalParameters.T8_delPw./mpc.dynamicdata.gen_pssParameters.pss_delPw_signalParameters.T9_delPw  SaturateOnIntegerOverflow=on  OutDataTypeStr=Inherit: Same as input  ParamDataTypeStr=Inherit: Same as input
  Integrator4 : Integrator
  Sum3 : Sum  SaturateOnIntegerOverflow=on  InputSameDT=on  OutDataTypeStr=Inherit: Same as first input
  Sum4 : Sum  Inputs=+-  SaturateOnIntegerOverflow=on  InputSameDT=on  OutDataTypeStr=Inherit: Same as first input
  Vs : Outport
  wires:
  Sum3/1 -> Vs/1
  in/1 -> Gain4/1, Gain5/1
  Gain4/1 -> Sum3/2
  Integrator4/1 -> Sum3/1, Sum4/2
  Gain3/1 -> Integrator4/1
  Sum4/1 -> Gain3/1
  Gain5/1 -> Sum4/1

== system transientStability_R2014B_SLX/PSS/delP_Omega_PSS/Filtering M=2 and N=4/Subsystem1/delay1 ==
  Vin : Inport
  Gain : Gain  Gain=1./mpc.dynamicdata.gen_pssParameters.pss_delPw_signalParameters.T9_delPw  SaturateOnIntegerOverflow=on  OutDataTypeStr=Inherit: Same as input  ParamDataTypeStr=Inherit: Same as input
  Integrator2 : Integrator
  Sum : Sum  Inputs=+-  SaturateOnIntegerOverflow=on  InputSameDT=on  OutDataTypeStr=Inherit: Same as first input
  Out1 : Outport
  wires:
  Gain/1 -> Integrator2/1
  Sum/1 -> Gain/1
  Integrator2/1 -> Out1/1, Sum/2
  Vin/1 -> Sum/1

== system transientStability_R2014B_SLX/PSS/delP_Omega_PSS/Filtering M=2 and N=4/Subsystem2/Compensator ==
  in : Inport
  Gain3 : Gain  Gain=1./mpc.dynamicdata.gen_pssParameters.pss_delPw_signalParameters.T9_delPw  SaturateOnIntegerOverflow=on  OutDataTypeStr=Inherit: Same as input  ParamDataTypeStr=Inherit: Same as input
  Gain4 : Gain  Gain=mpc.dynamicdata.gen_pssParameters.pss_delPw_signalParameters.T8_delPw./mpc.dynamicdata.gen_pssParameters.pss_delPw_signalParameters.T9_delPw  SaturateOnIntegerOverflow=on  OutDataTypeStr=Inherit: Same as input  ParamDataTypeStr=Inherit: Same as input
  Gain5 : Gain  Gain=1-mpc.dynamicdata.gen_pssParameters.pss_delPw_signalParameters.T8_delPw./mpc.dynamicdata.gen_pssParameters.pss_delPw_signalParameters.T9_delPw  SaturateOnIntegerOverflow=on  OutDataTypeStr=Inherit: Same as input  ParamDataTypeStr=Inherit: Same as input
  Integrator4 : Integrator
  Sum3 : Sum  SaturateOnIntegerOverflow=on  InputSameDT=on  OutDataTypeStr=Inherit: Same as first input
  Sum4 : Sum  Inputs=+-  SaturateOnIntegerOverflow=on  InputSameDT=on  OutDataTypeStr=Inherit: Same as first input
  Vs : Outport
  wires:
  Gain5/1 -> Sum4/1
  Sum4/1 -> Gain3/1
  Gain3/1 -> Integrator4/1
  Integrator4/1 -> Sum4/2, Sum3/1
  Gain4/1 -> Sum3/2
  in/1 -> Gain5/1, Gain4/1
  Sum3/1 -> Vs/1

== system transientStability_R2014B_SLX/PSS/delP_Omega_PSS/Filtering M=2 and N=4/Subsystem2/delay1 ==
  Vin : Inport
  Gain : Gain  Gain=1./mpc.dynamicdata.gen_pssParameters.pss_delPw_signalParameters.T9_delPw  SaturateOnIntegerOverflow=on  OutDataTypeStr=Inherit: Same as input  ParamDataTypeStr=Inherit: Same as input
  Integrator2 : Integrator
  Sum : Sum  Inputs=+-  SaturateOnIntegerOverflow=on  InputSameDT=on  OutDataTypeStr=Inherit: Same as first input
  Out1 : Outport
  wires:
  Vin/1 -> Sum/1
  Integrator2/1 -> Sum/2, Out1/1
  Sum/1 -> Gain/1
  Gain/1 -> Integrator2/1

== system transientStability_R2014B_SLX/PSS/delP_Omega_PSS/Filtering M=2 and N=4/Subsystem3/Compensator ==
  in : Inport
  Gain3 : Gain  Gain=1./mpc.dynamicdata.gen_pssParameters.pss_delPw_signalParameters.T9_delPw  SaturateOnIntegerOverflow=on  OutDataTypeStr=Inherit: Same as input  ParamDataTypeStr=Inherit: Same as input
  Gain4 : Gain  Gain=mpc.dynamicdata.gen_pssParameters.pss_delPw_signalParameters.T8_delPw./mpc.dynamicdata.gen_pssParameters.pss_delPw_signalParameters.T9_delPw  SaturateOnIntegerOverflow=on  OutDataTypeStr=Inherit: Same as input  ParamDataTypeStr=Inherit: Same as input
  Gain5 : Gain  Gain=1-mpc.dynamicdata.gen_pssParameters.pss_delPw_signalParameters.T8_delPw./mpc.dynamicdata.gen_pssParameters.pss_delPw_signalParameters.T9_delPw  SaturateOnIntegerOverflow=on  OutDataTypeStr=Inherit: Same as input  ParamDataTypeStr=Inherit: Same as input
  Integrator4 : Integrator
  Sum3 : Sum  SaturateOnIntegerOverflow=on  InputSameDT=on  OutDataTypeStr=Inherit: Same as first input
  Sum4 : Sum  Inputs=+-  SaturateOnIntegerOverflow=on  InputSameDT=on  OutDataTypeStr=Inherit: Same as first input
  Vs : Outport
  wires:
  Sum3/1 -> Vs/1
  in/1 -> Gain4/1, Gain5/1
  Gain4/1 -> Sum3/2
  Integrator4/1 -> Sum3/1, Sum4/2
  Gain3/1 -> Integrator4/1
  Sum4/1 -> Gain3/1
  Gain5/1 -> Sum4/1

== system transientStability_R2014B_SLX/PSS/delP_Omega_PSS/Filtering M=2 and N=4/Subsystem3/delay1 ==
  Vin : Inport
  Gain : Gain  Gain=1./mpc.dynamicdata.gen_pssParameters.pss_delPw_signalParameters.T9_delPw  SaturateOnIntegerOverflow=on  OutDataTypeStr=Inherit: Same as input  ParamDataTypeStr=Inherit: Same as input
  Integrator2 : Integrator
  Sum : Sum  Inputs=+-  SaturateOnIntegerOverflow=on  InputSameDT=on  OutDataTypeStr=Inherit: Same as first input
  Out1 : Outport
  wires:
  Gain/1 -> Integrator2/1
  Sum/1 -> Gain/1
  Integrator2/1 -> Out1/1, Sum/2
  Vin/1 -> Sum/1

== system transientStability_R2014B_SLX/PSS/frequency_input_PSS /delta_Freq/derivative1/1//1+s*Tf ==
  In1 : Inport
  1/Tf : Gain  Gain=[1./0.02]  SaturateOnIntegerOverflow=on  OutDataTypeStr=Inherit: Same as input  ParamDataTypeStr=Inherit: Same as input
  In2 : Integrator  InitialCondition=imag(mpc.dynamicdata.Vpre(mpc.dynamicdata.freq_pss(:,1)))
  Sum3 : Sum  Inputs=+-  SaturateOnIntegerOverflow=on  InputSameDT=on  OutDataTypeStr=Inherit: Same as first input
  Out1 : Outport
  wires:
  Sum3/1 -> 1/Tf/1
  1/Tf/1 -> In2/1
  In2/1 -> Sum3/2, Out1/1
  In1/1 -> Sum3/1

== system transientStability_R2014B_SLX/PSS/frequency_input_PSS /delta_Freq/derivative2/1//1+s*Tf ==
  In1 : Inport
  1/Tf : Gain  Gain=[1./0.02]  SaturateOnIntegerOverflow=on  OutDataTypeStr=Inherit: Same as input  ParamDataTypeStr=Inherit: Same as input
  In2 : Integrator  InitialCondition=real(mpc.dynamicdata.Vpre(mpc.dynamicdata.freq_pss(:,1)))
  Sum3 : Sum  Inputs=+-  SaturateOnIntegerOverflow=on  InputSameDT=on  OutDataTypeStr=Inherit: Same as first input
  Out1 : Outport
  wires:
  In2/1 -> Out1/1, Sum3/2
  1/Tf/1 -> In2/1
  Sum3/1 -> 1/Tf/1
  In1/1 -> Sum3/1
